simulink subsystem "Generator"  (R2024a)
settings: Solver=VariableStepAuto  StartTime=0.0  StopTime=10.0  RelTol=1e-3
PreLoadFcn:
  | k_e = 5.4e-3;
  | R_a = 1.94e-3;
  | L = 77e-6;
settings Model: Creator=User  LastModifiedBy=User

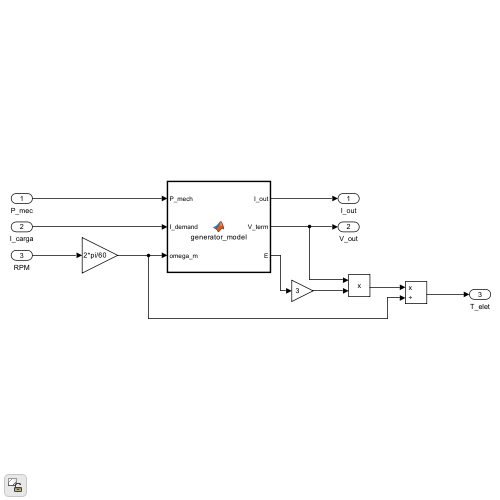
[thumbnail: Simulink's stored preview of the top-level diagram]
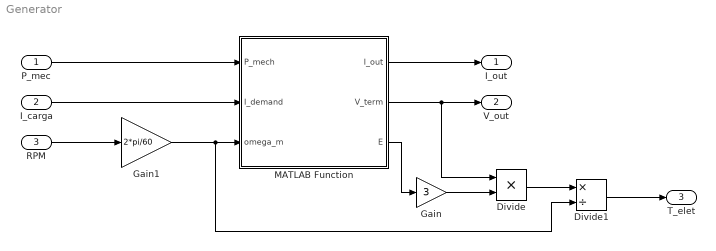
== system Generator ==
  P_mec : Inport
  I_carga : Inport  Port=2
  RPM : Inport  Port=3
  Divide : Product  Inputs=**
  Divide1 : Product  Inputs=*/
  Gain : Gain  Gain=3
  Gain1 : Gain  Gain=2*pi/60
  MATLAB Function : MATLAB Function  TreatAsAtomicUnit=on
  I_out : Outport
  V_out : Outport  Port=2
  T_elet : Outport  Port=3
  wires:
  P_mec/1 -> MATLAB Function/1(P_mech)
  I_carga/1 -> MATLAB Function/2(I_demand)
  MATLAB Function/1(I_out) -> I_out/1
  MATLAB Function/2(V_term) -> Divide/1, V_out/1
  MATLAB Function/3(E) -> Gain/1
  Gain/1 -> Divide/2
  Divide/1 -> Divide1/1
  RPM/1 -> Gain1/1
  Divide1/1 -> T_elet/1
  Gain1/1 -> Divide1/2, MATLAB Function/3(omega_m)

== matlab function Generator/MATLAB Function ==
  data: P_mech input; I_out output; I_demand input; omega_m input; V_term output; E output
function [I_out, V_term, E] = generator_model(P_mech, I_demand, omega_m)
    % Parâmetros do gerador
    Ra = 1.94e-3;      % Resistência de armadura [Ω]
    Ls = 77e-6;        % Indutância síncrona [H]
    k = 5.4e-3;        % Constante de tensão [V/rpm]
    poles = 10;        % Número de polos
    
    % Conversão de velocidade mecânica para elétrica
    omega_e = (poles/2) * omega_m * (2*pi/60); % [rad/s]
    
    % Força eletromotriz (FEM) induzida
    E = k * omega_m;   % FEM por fase [V]
    
    % Considerando operação em regime permanente
    
    % Impedância síncrona
    Zs = Ra + 1j*omega_e*Ls;
    
    % Corrente calculada baseada no balanço de potência
    P_elec = P_mech - mechanical_losses(omega_m); % Considerar perdas mecânicas
    I_calc = P_elec / (3*E); % Corrente aproximada
    
    % Limitar pela corrente exigida
    I_out = min(I_calc, I_demand);
    
    % Tensão terminal
    V_term = E - Zs*I_out;
end
